simulink model "uncontrolledRectifier"  (R2021a)
settings: Solver=ode23t  StartTime=0.0  StopTime=.1  FixedStep=.000001  MaxStep=.0001  RelTol=1e-3
undefined symbols (not defined in the file): D1, D11, Delta
libraries: spsDiodeLib x39, spsVoltageMeasurementLib x37, spsACVoltageSourceLib x17, spsCurrentMeasurementLib x13, spsSeriesRLCBranchLib x10, spsGroundLib x2, spsThreePhaseTransformerThreeWindingsLib x1, spspowerguiLib x1
settings Model: Creator=User  LastModifiedBy=User

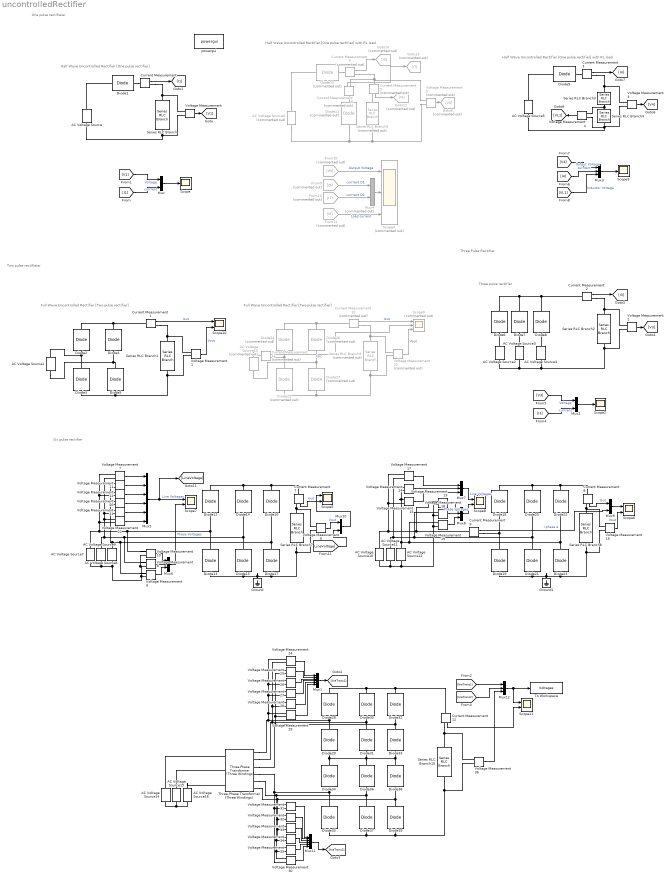
== system uncontrolledRectifier ==
  note: Six pulse rectifier
  note: Three Pulse Rectifier
  note: Two pulse rectifieier
  note: One pulse rectifieier
  note: Three pulse rectifier
  note: Half Wave Uncontrolled Rectifier [One pulse rectifier]
  note: Full Wave Uncontrolled Rectifier [Two pulse rectifier]
  note: Half Wave Uncontrolled Rectifier [One pulse rectifier] with RL load
  note: Half Wave Uncontrolled Rectifier [One pulse rectifier] with RL load
  note: Full Wave Uncontrolled Rectifier [Two pulse rectifier]
  AC Voltage Source{,1..2,5,7,10} (6 alike) : spsACVoltageSourceLib/AC Voltage Source  Amplitude=220  Phase=0  Frequency=50  SampleTime=0  Measurements=None  BusType=swing  Pref=10e3  Qref=0  Qmin=-inf  Qmax=+inf
  AC Voltage Source11 : spsACVoltageSourceLib/AC Voltage Source  Amplitude=220  Phase=-120  Frequency=50  SampleTime=0  Measurements=None  BusType=swing  Pref=10e3  Qref=0  Qmin=-inf  Qmax=+inf
  AC Voltage Source12 : spsACVoltageSourceLib/AC Voltage Source  Amplitude=220  Phase=120  Frequency=50  SampleTime=0  Measurements=None  BusType=swing  Pref=10e3  Qref=0  Qmin=-inf  Qmax=+inf
  AC Voltage Source13 : spsACVoltageSourceLib/AC Voltage Source  Commented=on  Amplitude=220  Phase=0  Frequency=50  SampleTime=0  Measurements=None  BusType=swing  Pref=10e3  Qref=0  Qmin=-inf  Qmax=+inf
  AC Voltage Source14 : spsACVoltageSourceLib/AC Voltage Source  Amplitude=220*sqrt(2)  Phase=0  Frequency=50  SampleTime=0  Measurements=None  BusType=swing  Pref=10e3  Qref=0  Qmin=-inf  Qmax=+inf
  AC Voltage Source15 : spsACVoltageSourceLib/AC Voltage Source  Amplitude=220*sqrt(2)  Phase=-120  Frequency=50  SampleTime=0  Measurements=None  BusType=swing  Pref=10e3  Qref=0  Qmin=-inf  Qmax=+inf
  AC Voltage Source16 : spsACVoltageSourceLib/AC Voltage Source  Amplitude=220*sqrt(2)  Phase=120  Frequency=50  SampleTime=0  Measurements=None  BusType=swing  Pref=10e3  Qref=0  Qmin=-inf  Qmax=+inf
  AC Voltage Source3 : spsACVoltageSourceLib/AC Voltage Source  Amplitude=220  Phase=120  Frequency=50  SampleTime=0  Measurements=None  BusType=swing  Pref=10e3  Qref=0  Qmin=-inf  Qmax=+inf
  AC Voltage Source4 : spsACVoltageSourceLib/AC Voltage Source  Amplitude=220  Phase=240  Frequency=50  SampleTime=0  Measurements=None  BusType=swing  Pref=10e3  Qref=0  Qmin=-inf  Qmax=+inf
  AC Voltage Source6 : spsACVoltageSourceLib/AC Voltage Source  Commented=on  Amplitude=220  Phase=0  Frequency=50  SampleTime=0  Measurements=None  BusType=swing  Pref=10e3  Qref=0  Qmin=-inf  Qmax=+inf
  AC Voltage Source8 : spsACVoltageSourceLib/AC Voltage Source  Amplitude=220  Phase=-120  Frequency=50  SampleTime=0  Measurements=None  BusType=swing  Pref=10e3  Qref=0  Qmin=-inf  Qmax=+inf
  AC Voltage Source9 : spsACVoltageSourceLib/AC Voltage Source  Amplitude=220  Phase=120  Frequency=50  SampleTime=0  Measurements=None  BusType=swing  Pref=10e3  Qref=0  Qmin=-inf  Qmax=+inf
  Current Measurement{,1..3,7..9,12} (8 alike) : spsCurrentMeasurementLib/Current Measurement  PhasorSimulation=off  OutputType=Complex  PSBequivalent=0
  Current Measurement{4..6,10..11} (5 alike) : spsCurrentMeasurementLib/Current Measurement  Commented=on  PhasorSimulation=off  OutputType=Complex  PSBequivalent=0
  Diode{1..9,12..23,28..39} (33 alike) : spsDiodeLib/Diode  Ron=0.001  Lon=0  Vf=0.8  IC=0  UseSnubber=0  Rs=500  Cs=250e-9  Measurements=off
  Diode{10..11,24..27} (6 alike) : spsDiodeLib/Diode  Commented=on  Ron=0.001  Lon=0  Vf=0.8  IC=0  UseSnubber=0  Rs=500  Cs=250e-9  Measurements=off
  From10 : From  Commented=on  GotoTag=V5
  From12 : From  Commented=on  GotoTag=I6
  From13 : From  Commented=on  GotoTag=I7
  From9 : From  Commented=on  GotoTag=I5
  Goto10 : Goto  Commented=on  GotoTag=I5
  Goto12 : Goto  Commented=on  GotoTag=I6
  Goto13 : Goto  Commented=on  GotoTag=I7
  Goto9 : Goto  Commented=on  GotoTag=V5
  Ground : spsGroundLib/Ground  LConnTagsString=a
  Ground1 : spsGroundLib/Ground  LConnTagsString=a
  Mux{,2,9..10} (4 alike) : Mux  Inputs=2
  Mux1 : Mux  Inputs=6
  Mux11 : Mux  Inputs=6
  Mux{3,6..8,12} (5 alike) : Mux  Inputs=3
  Mux4 : Mux  Commented=on  Inputs=2
  Mux5 : Mux  Inputs=6
  Scope : Scope
  Scope{5..8,10..11} (6 alike) : Scope  NumInputPorts=2
  Scope2 : Scope
  Scope3 : Scope
  Scope4 : Scope  Commented=on  NumInputPorts=3
  Scope9 : Scope  Commented=on  NumInputPorts=3
  Series RLC Branch{,1..3,7,10} (6 alike) : spsSeriesRLCBranchLib/Series RLC Branch  LConnTagsString=__new0  RConnTagsString=__new0  BranchType=R  Resistance=10  Inductance=1e-3  SetiL0=off  InitialCurrent=0  Capacitance=1e-6  Setx0=off  InitialVoltage=0  Measurements=None
  Series RLC Branch4 : spsSeriesRLCBranchLib/Series RLC Branch  LConnTagsString=__new0  RConnTagsString=__new0  BranchType=L  Resistance=10  Inductance=10/(2*pi*50)  SetiL0=off  InitialCurrent=0  Capacitance=1e-6  Setx0=off  InitialVoltage=0  Measurements=None
  Series RLC Branch5 : spsSeriesRLCBranchLib/Series RLC Branch  Commented=on  LConnTagsString=__new0  RConnTagsString=__new0  BranchType=RL  Resistance=10  Inductance=1  SetiL0=off  InitialCurrent=0  Capacitance=1e-6  Setx0=off  InitialVoltage=0  Measurements=None
  Series RLC Branch8 : spsSeriesRLCBranchLib/Series RLC Branch  LConnTagsString=__new0  RConnTagsString=__new0  BranchType=RL  Resistance=10  Inductance=100e-3  SetiL0=off  InitialCurrent=0  Capacitance=1e-6  Setx0=off  InitialVoltage=0  Measurements=None
  Series RLC Branch9 : spsSeriesRLCBranchLib/Series RLC Branch  Commented=on  LConnTagsString=__new0  RConnTagsString=__new0  BranchType=RL  Resistance=10  Inductance=100e-3  SetiL0=off  InitialCurrent=0  Capacitance=1e-6  Setx0=off  InitialVoltage=0  Measurements=None
  Three-Phase Transformer (Three Windings) : spsThreePhaseTransformerThreeWindingsLib/Three-Phase Transformer (Three Windings)  Winding1Connection=Delta (D1)  Winding2Connection=Y  Winding3Connection=Delta (D11)  CoreType=Three single-phase transformers  SetSaturation=off  Hysteresis=off  DataFile='hysteresis'  SetInitialFlux=off  Measurements=None  UNITS=pu  NominalPower=[ 6000 , 50 ]  Winding1=[ 380 , 0.002 , 0.08 ]  Winding2=[ 100 , 0.002 , 0.08 ]  Winding3=[ 100 , 0.002 , 0.08 ]  Rm=500  Lm=500  L0=0.5  Saturation=[ 0,0 ; 0.0024,1.2 ; 1.0,1.52 ]  InitialFluxes=[0.8 -0.8 0.7]  BreakLoop=off  DiscreteSolver=Trapezoidal iterative  DataType=off  TransfoNumber=1
      settings: SourceProductBaseCode=PS
  To Workspace : ToWorkspace  VariableName=Voltages  SaveFormat=Structure With Time  SampleTime=-1
  Voltage Measurement{,1..4,6..22,24..36} (35 alike) : spsVoltageMeasurementLib/Voltage Measurement  PhasorSimulation=off  OutputType=Complex  PSBequivalent=0
  Voltage Measurement23 : spsVoltageMeasurementLib/Voltage Measurement  Commented=on  PhasorSimulation=off  OutputType=Complex  PSBequivalent=0
  Voltage Measurement5 : spsVoltageMeasurementLib/Voltage Measurement  Commented=on  PhasorSimulation=off  OutputType=Complex  PSBequivalent=0
  powergui : spspowerguiLib/powergui  Priority=1  SimulationMode=Continuous  SampleTime=50e-6  frequency=60  Iterations=50  frequencyindice=50  Pbase=100e6  ErrMax=1e-4  UnitsV=kV  UnitsW=MW  buscounter=0  FunctionMessages=off  echomessages=off  EnableUseOfTLC=off  CurrentSourceSwitches=off  DisableSnubberDevices=off  DisableRonSwitches=on  DisableVfSwitches=on  DisplayEquations=off  AutomaticDiscreteSolvers=off  SolverType=Tustin/Backward Euler (TBE)  Interpol=off  ExternalGateDelay=off  methode=off  Ts=100  x0status=blocks  SPID=on  SwTol=0  HookPort=off  NonlinearTolerance=1e-4  nMaxIteration=100  ContinueOnMaxIteration=off  RestoreLinks=warning  ResistiveCurrentMeasurement=off  Frange=[0:2:500]  Ylog=off  Xlog=on  ShowGrid=off  save=off  variable=ZData  structure=0  ZoomFFT=off  StartTime=0.0  cycles=1  DisplayStyle=1  fundamental=60  FreqAxis=off  MaxFrequency=1000  frequencyindicesteady=1  RmsSteady=1  display=off
  wires:
  Voltage Measurement/1 -> [V1]
  Current Measurement/1 -> [I1]
  [V1] -> Mux/1  "Voltage"
  [I1] -> Mux/2  "currrent"
  Mux/1 -> Scope/1
  Current Measurement1/1 -> Scope10/1  "Iout"
  Voltage Measurement1/1 -> Scope10/2  "Vout"
  Voltage Measurement2/1 -> [V3]
  Current Measurement2/1 -> [I3]
  [V3] -> Mux2/1  "Voltage"
  [I3] -> Mux2/2  "currrent"
  Mux2/1 -> Scope2/1
  Mux3/1 -> Scope3/1
  [I4] -> Mux3/2  "currrent"
  [V4] -> Mux3/1  "Output Voltage"
  Current Measurement3/1 -> [I4]
  Voltage Measurement3/1 -> [V4]
  Voltage Measurement4/1 -> [VL1]
  [VL1] -> Mux3/3  "Inductor Voltage"
  Voltage Measurement5/1 -> Goto9/1
  Current Measurement4/1 -> Goto10/1
  From10/1 -> Scope4/1  "Output Voltage"
  From9/1 -> Mux4/1  "currrent D1"
  Current Measurement5/1 -> Goto12/1
  From12/1 -> Scope4/3  "Load current"
  Current Measurement6/1 -> Goto13/1
  From13/1 -> Mux4/2  "currrent D2"
  Mux4/1 -> Scope4/2
  Current Measurement7/1 -> Scope5/2  "Iout"
  Voltage Measurement6/1 -> Mux10/1  "Vout"
  Voltage Measurement7/1 -> Mux5/1
  Voltage Measurement8/1 -> Mux6/2
  Voltage Measurement9/1 -> Mux6/3
  Voltage Measurement10/1 -> Mux6/1
  Voltage Measurement12/1 -> Mux5/3
  Voltage Measurement11/1 -> Mux5/2
  Mux5/1 -> [LineVoltage], Scope7/1  "Line Voltages"
  Mux6/1 -> Scope7/2  "Phase Voltages"
  Mux8/1 -> Scope8/2  "Phase Voltages"
  Mux7/1 -> Scope8/1  "Line Voltages"
  Voltage Measurement14/1 -> Mux7/2
  Voltage Measurement15/1 -> Mux7/3
  Voltage Measurement13/1 -> Mux8/1
  Voltage Measurement19/1 -> Mux8/3
  Voltage Measurement18/1 -> Mux8/2
  Voltage Measurement17/1 -> Mux7/1
  Voltage Measurement16/1 -> Scope6/2  "Vout"
  Current Measurement8/1 -> Mux9/1  "Iout"
  Current Measurement9/1 -> Mux9/2  "I phase a"
  Mux9/1 -> Scope6/1
  Voltage Measurement20/1 -> Mux5/4
  Voltage Measurement21/1 -> Mux5/5
  Voltage Measurement22/1 -> Mux5/6
  Mux10/1 -> Scope5/1
  [LineVoltage] -> Mux10/2
  Voltage Measurement23/1 -> Scope9/3  "Vout"
  Current Measurement10/1 -> Scope9/1  "Iout"
  Current Measurement11/1 -> Scope9/2  "Isrc"
  Voltage Measurement24/1 -> Mux1/1
  Voltage Measurement25/1 -> Mux1/2
  Voltage Measurement26/1 -> Mux1/3
  Voltage Measurement27/1 -> Mux1/4
  Voltage Measurement28/1 -> Mux1/5
  Voltage Measurement29/1 -> Mux1/6
  Mux1/1 -> [lineTrans1]
  Mux11/1 -> [lineTrans2]
  Voltage Measurement30/1 -> Mux11/6
  Voltage Measurement35/1 -> Mux11/5
  Voltage Measurement34/1 -> Mux11/4
  Voltage Measurement33/1 -> Mux11/3
  Voltage Measurement32/1 -> Mux11/2
  Voltage Measurement31/1 -> Mux11/1
  [lineTrans1] -> Mux12/1
  [lineTrans2] -> Mux12/2
  Voltage Measurement36/1 -> Mux12/3
  Current Measurement12/1 -> Scope11/2
  Mux12/1 -> To Workspace/1, Scope11/1
  connections:
  Diode1/LConn1 -- AC Voltage Source/RConn1
  Voltage Measurement/LConn1 -- Current Measurement/RConn1 -- Series RLC Branch/LConn1
  AC Voltage Source/LConn1 -- Voltage Measurement/LConn2 -- Series RLC Branch/RConn1
  Diode1/RConn1 -- Current Measurement/LConn1
  Current Measurement1/RConn1 -- Voltage Measurement1/LConn1 -- Series RLC Branch1/LConn1
  Voltage Measurement1/LConn2 -- Diode3/LConn1 -- Diode5/LConn1 -- Series RLC Branch1/RConn1
  Diode2/RConn1 -- Diode4/RConn1 -- Current Measurement1/LConn1
  Diode3/RConn1 -- AC Voltage Source1/RConn1 -- Diode2/LConn1
  Diode5/RConn1 -- AC Voltage Source1/LConn1 -- Diode4/LConn1
  Voltage Measurement2/LConn1 -- Current Measurement2/RConn1 -- Series RLC Branch2/LConn1
  Voltage Measurement2/LConn2 -- AC Voltage Source2/LConn1 -- AC Voltage Source3/LConn1 -- AC Voltage Source4/LConn1 -- Series RLC Branch2/RConn1
  Diode8/RConn1 -- Diode7/RConn1 -- Diode6/RConn1 -- Current Measurement2/LConn1
  AC Voltage Source2/RConn1 -- Diode6/LConn1
  AC Voltage Source3/RConn1 -- Diode7/LConn1
  AC Voltage Source4/RConn1 -- Diode8/LConn1
  Current Measurement3/RConn1 -- Voltage Measurement3/LConn1 -- Series RLC Branch3/LConn1
  AC Voltage Source5/LConn1 -- Voltage Measurement4/LConn2 -- Voltage Measurement3/LConn2 -- Series RLC Branch4/RConn1
  Diode9/RConn1 -- Current Measurement3/LConn1
  Diode9/LConn1 -- AC Voltage Source5/RConn1
  Series RLC Branch4/LConn1 -- Voltage Measurement4/LConn1 -- Series RLC Branch3/RConn1
  Current Measurement4/RConn1 -- Current Measurement5/LConn1 -- Voltage Measurement5/LConn1 -- Current Measurement6/RConn1
  Voltage Measurement5/LConn2 -- Diode11/LConn1 -- AC Voltage Source6/LConn1 -- Series RLC Branch5/RConn1
  Diode10/LConn1 -- AC Voltage Source6/RConn1
  Diode10/RConn1 -- Current Measurement4/LConn1
  Current Measurement5/RConn1 -- Series RLC Branch5/LConn1
  Current Measurement6/LConn1 -- Diode11/RConn1
  Diode15/LConn1 -- Diode13/LConn1 -- Ground/LConn1 -- Voltage Measurement6/LConn2 -- Series RLC Branch7/RConn1 -- Diode17/LConn1
  Series RLC Branch7/LConn1 -- Voltage Measurement6/LConn1 -- Current Measurement7/RConn1
  AC Voltage Source8/RConn1 -- Voltage Measurement22/LConn1 -- Voltage Measurement7/LConn2 -- Voltage Measurement11/LConn1 -- Voltage Measurement21/LConn2 -- Diode15/RConn1 -- Diode14/LConn1 -- Voltage Measurement8/LConn1
  AC Voltage Source7/RConn1 -- Voltage Measurement22/LConn2 -- Voltage Measurement12/LConn2 -- Voltage Measurement7/LConn1 -- Voltage Measurement20/LConn1 -- Diode12/LConn1 -- Diode13/RConn1 -- Voltage Measurement10/LConn1
  AC Voltage Source9/RConn1 -- Voltage Measurement20/LConn2 -- Voltage Measurement12/LConn1 -- Voltage Measurement11/LConn2 -- Voltage Measurement21/LConn1 -- Diode16/LConn1 -- Diode17/RConn1 -- Voltage Measurement9/LConn1
  AC Voltage Source8/LConn1 -- AC Voltage Source9/LConn1 -- Voltage Measurement10/LConn2 -- Voltage Measurement8/LConn2 -- Voltage Measurement9/LConn2 -- AC Voltage Source7/LConn1
  Current Measurement7/LConn1 -- Diode14/RConn1 -- Diode12/RConn1 -- Diode16/RConn1
  Diode21/LConn1 -- Diode23/LConn1 -- Series RLC Branch8/RConn1 -- Voltage Measurement16/LConn2 -- Ground1/LConn1 -- Diode19/LConn1
  Series RLC Branch8/LConn1 -- Current Measurement8/RConn1 -- Voltage Measurement16/LConn1
  Voltage Measurement17/LConn2 -- Voltage Measurement14/LConn1 -- AC Voltage Source11/RConn1 -- Voltage Measurement18/LConn1 -- Diode20/LConn1 -- Diode21/RConn1
  Diode19/RConn1 -- Diode18/LConn1 -- Current Measurement9/RConn1
  Voltage Measurement15/LConn1 -- Voltage Measurement14/LConn2 -- AC Voltage Source12/RConn1 -- Voltage Measurement19/LConn1 -- Diode23/RConn1 -- Diode22/LConn1
  AC Voltage Source12/LConn1 -- Voltage Measurement19/LConn2 -- Voltage Measurement18/LConn2 -- Voltage Measurement13/LConn2 -- AC Voltage Source11/LConn1 -- AC Voltage Source10/LConn1
  Current Measurement8/LConn1 -- Diode22/RConn1 -- Diode18/RConn1 -- Diode20/RConn1
  Voltage Measurement15/LConn2 -- Voltage Measurement17/LConn1 -- AC Voltage Source10/RConn1 -- Voltage Measurement13/LConn1 -- Current Measurement9/LConn1
  Current Measurement10/RConn1 -- Series RLC Branch9/LConn1 -- Voltage Measurement23/LConn1
  Voltage Measurement23/LConn2 -- Series RLC Branch9/RConn1 -- Diode27/LConn1 -- Diode25/LConn1
  Diode24/RConn1 -- Current Measurement10/LConn1 -- Diode26/RConn1
  AC Voltage Source13/RConn1 -- Current Measurement11/LConn1
  Diode27/RConn1 -- Diode26/LConn1 -- AC Voltage Source13/LConn1
  Current Measurement11/RConn1 -- Diode24/LConn1 -- Diode25/RConn1
  Diode29/RConn1 -- Voltage Measurement29/LConn1 -- Voltage Measurement28/LConn1 -- Voltage Measurement27/LConn2 -- Voltage Measurement26/LConn2 -- Voltage Measurement24/LConn1 -- Three-Phase Transformer (Three Windings)/RConn1 -- Diode28/LConn1
  Diode31/RConn1 -- Voltage Measurement28/LConn2 -- Voltage Measurement27/LConn1 -- Voltage Measurement24/LConn2 -- Voltage Measurement25/LConn1 -- Three-Phase Transformer (Three Windings)/RConn2 -- Diode30/LConn1
  Diode33/RConn1 -- Voltage Measurement29/LConn2 -- Voltage Measurement25/LConn2 -- Voltage Measurement26/LConn1 -- Three-Phase Transformer (Three Windings)/RConn3 -- Diode32/LConn1
  Diode30/RConn1 -- Current Measurement12/LConn1 -- Diode32/RConn1 -- Diode28/RConn1
  Diode35/LConn1 -- Diode37/LConn1 -- Voltage Measurement36/LConn2 -- Series RLC Branch10/RConn1 -- Diode39/LConn1
  Diode37/RConn1 -- Three-Phase Transformer (Three Windings)/RConn5 -- Voltage Measurement33/LConn1 -- Voltage Measurement35/LConn2 -- Voltage Measurement30/LConn1 -- Voltage Measurement34/LConn2 -- Diode36/LConn1
  Diode35/RConn1 -- Voltage Measurement32/LConn1 -- Voltage Measurement35/LConn1 -- Voltage Measurement30/LConn2 -- Voltage Measurement31/LConn2 -- Three-Phase Transformer (Three Windings)/RConn4 -- Diode34/LConn1
  Diode39/RConn1 -- Voltage Measurement31/LConn1 -- Voltage Measurement32/LConn2 -- Voltage Measurement33/LConn2 -- Voltage Measurement34/LConn1 -- Three-Phase Transformer (Three Windings)/RConn6 -- Diode38/LConn1
  AC Voltage Source15/LConn1 -- AC Voltage Source16/LConn1 -- AC Voltage Source14/LConn1
  AC Voltage Source14/RConn1 -- Three-Phase Transformer (Three Windings)/LConn1
  AC Voltage Source15/RConn1 -- Three-Phase Transformer (Three Windings)/LConn2
  AC Voltage Source16/RConn1 -- Three-Phase Transformer (Three Windings)/LConn3
  Diode36/RConn1 -- Diode34/RConn1 -- Diode29/LConn1 -- Diode31/LConn1 -- Diode33/LConn1 -- Diode38/RConn1
  Current Measurement12/RConn1 -- Voltage Measurement36/LConn1 -- Series RLC Branch10/LConn1
